simulink model "AxisIntegratorTest"  (R2016a)
settings: Solver=VariableStepAuto  StartTime=0.0  StopTime=10.0  RelTol=1e-3
libraries: SimscapeMacros x3, ProjectBlocks x2, fl_lib x1, nesl_utility x1
settings Model: Creator=Peter  LastModifiedBy=Peter

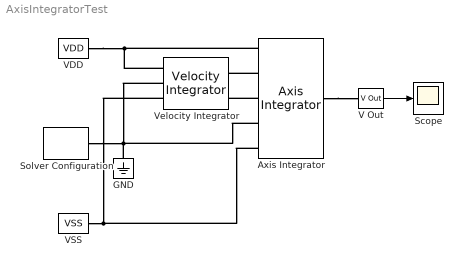
== system AxisIntegratorTest ==
  Axis Integrator : ProjectBlocks/Axis Integrator
  GND : fl_lib/Electrical/Electrical Elements/Electrical Reference
  Scope : Scope
  Solver Configuration : nesl_utility/Solver Configuration  PhysicalDomain=network_engine_domain  SubClassName=solver  LeftPortType=input  RightPortType=generic  Accelerate=off  Tones=[]  Harmonics=[]  SimulateNoise=off  Profile=off  UseLocalSampling=off  EnableSwitchedLinearOptims=on  FrequencyDomain=off  UseCCode=off  RelTol=0.001  AbsTol=1e-06  MinStep=1e-09  ToWorkspace=off  RevertToSquareIcSolve=off  NumHomotopyIterations=100  PhasorMode=off  PhasorModeNumHarmonics=1  OverrideAbsTol=off  DoDC=off  ResidualTolerance=1e-09  UseLocalSolver=off  LocalSolverChoice=NE_BACKWARD_EULER_ADVANCER  LocalSolverSampleTime=0.001  DoFixedCost=off  MaxNonlinIter=3  MaxModeIter=2  LinearAlgebra=Sparse  DelaysMemoryBudget=1024  AutomaticFiltering=on  FilteringTimeConstant=0.001
  V Out : SimscapeMacros/V Out
  VDD : SimscapeMacros/VDD
  VSS : SimscapeMacros/VSS
  Velocity Integrator : ProjectBlocks/Velocity Integrator
  wires:
  V Out/1 -> Scope/1
  connections:
  VDD/RConn1 -- Axis Integrator/LConn1 -- Velocity Integrator/LConn1
  GND/LConn1 -- Axis Integrator/LConn4 -- Solver Configuration/RConn1 -- Velocity Integrator/LConn2
  VSS/RConn1 -- Axis Integrator/LConn5 -- Velocity Integrator/LConn3
  Axis Integrator/LConn3 -- Velocity Integrator/RConn2
  Axis Integrator/LConn2 -- Velocity Integrator/RConn1
  Axis Integrator/RConn1 -- V Out/LConn1
